simulink model "part_5"  (R2025b)
settings: Solver=VariableStepAuto  StartTime=0.0  StopTime=10.0  RelTol=1e-3
libraries: dspxfrm3 x1
settings Model: Creator=Ultor  LastModifiedBy=Ultor

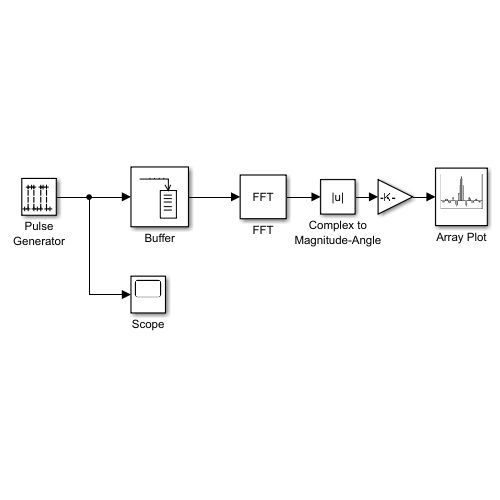
[thumbnail: Simulink's stored preview of the top-level diagram]
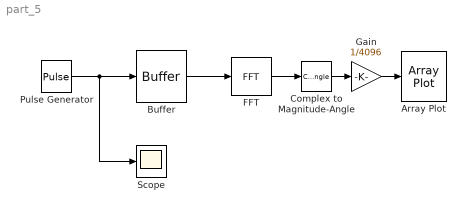
== system part_5 ==
  Array Plot : ArrayPlot  WindowPosition=[0.000000,36.000000,1920.000000,1009.000000,]  Visible=on  ScopeFrameLocation=window  YLimits=[-0.0097 0.0873]
  Buffer : Buffer  N=4096  OutputFrames=off
  Complex to Magnitude-Angle : ComplexToMagnitudeAngle  Output=Magnitude
  FFT : dspxfrm3/FFT  FFTImplementation=Auto  CompMethod=Table lookup  TableOpt=NEW  TableOptActive=Speed  BitRevOrder=off  Normalize=off  InheritFFTLength=on  FFTLength=64  WrapInput=on  roundingMode=Ceiling  overflowMode=off  firstCoeffDataTypeStr=Inherit: Same word length as input  firstCoeffLastDataTypeStr=Inherit: Same word length as input  outputMin=[]  outputMax=[]
  Gain : Gain  Gain=1/4096
  Pulse Generator : DiscretePulseGenerator  Period=8800  PulseWidth=440  SampleTime=1/440
  Scope : Scope
      settings: ActiveDisplayYMinimum=-0.12499999999999997  ActiveDisplayYMaximum=1.125
  wires:
  Pulse Generator/1 -> Scope/1, Buffer/1
  Buffer/1 -> FFT/1
  Complex to Magnitude-Angle/1 -> Gain/1
  FFT/1 -> Complex to Magnitude-Angle/1
  Gain/1 -> Array Plot/1
